simulink model "DecentralizedLFADRC"  (R2018a)
settings: Solver=ode4  StartTime=0.0  StopTime=480  FixedStep=1e-3  MaxStep=1e-4  RelTol=1e-3  EnableMultiTasking=on
values from neighbouring files (symbols this model uses):
  a_1 = 0.5    [DecentralizedADRC.m]
  a_10 = 0.125    [DecentralizedADRC.m]
  a_2 = 0.125    [DecentralizedADRC.m]
  a_3 = 0.125    [DecentralizedADRC.m]
  a_4 = 0.5    [DecentralizedADRC.m]
  a_5 = 0.1    [DecentralizedADRC.m]
  a_6 = 0.1    [DecentralizedADRC.m]
  a_7 = 0.1    [DecentralizedADRC.m]
  a_8 = 0.125    [DecentralizedADRC.m]
  a_9 = 0.5    [DecentralizedADRC.m]
  a_PV1 = 0.125    [DecentralizedADRC.m]
  a_PV2 = 0.2    [DecentralizedADRC.m]
  a_PV3 = 0.125    [DecentralizedADRC.m]
  a_WT1 = 0.125    [DecentralizedADRC.m]
  a_WT3 = 0.125    [DecentralizedADRC.m]
  B1 = (1/Req1)+D    [DecentralizedADRC.m]
  B2 = (1/Req2)+D    [DecentralizedADRC.m]
  B3 = (1/Req3)+D    [DecentralizedADRC.m]
  D = 2    [DecentralizedADRC.m]
  H_A1 = (H1*S1+H2*S2+H3*S3)/(S1+S2+S3)    (= 2.58715528865)    [DecentralizedADRC.m]
  H_A2 = (H4*S4+H5*S5+H6*S6+H7*S7)/(S4+S5+S6+S7)    (= 2.6419)    [DecentralizedADRC.m]
  H_A3 = (H8*S8+H9*S9+H10*S10)/(S8+S9+S10)    (= 2.49952427226)    [DecentralizedADRC.m]
  K1 = -K1    [DecentralizedADRC.m]
  K2 = -K2    [DecentralizedADRC.m]
  K3 = -K3    [DecentralizedADRC.m]
  kpc = 0.8    [DecentralizedADRC.m]
  R1 = 0.0548    [DecentralizedADRC.m]
  R4 = 0.06    [DecentralizedADRC.m]
  R9 = 0.0548    [DecentralizedADRC.m]
  Rp10 = 0.06    [DecentralizedADRC.m]
  Rp2 = 0.06    [DecentralizedADRC.m]
  Rp3 = 0.06    [DecentralizedADRC.m]
  Rp5 = 0.0548    [DecentralizedADRC.m]
  Rp6 = 0.06    [DecentralizedADRC.m]
  Rp7 = 0.06    [DecentralizedADRC.m]
  Rp8 = 0.06    [DecentralizedADRC.m]
  RPV1 = 0.05    [DecentralizedADRC.m]
  RPV2 = 0.05    [DecentralizedADRC.m]
  RPV3 = 0.05    [DecentralizedADRC.m]
  RWT1 = 0.024    [DecentralizedADRC.m]
  RWT3 = 0.024    [DecentralizedADRC.m]
  T12 = 2.5    [DecentralizedADRC.m]
  T13 = 5.0    (= 5)    [DecentralizedADRC.m]
  T23 = 3.8    [DecentralizedADRC.m]
undefined symbols (not defined in the file or in its folder): A_obs_1, A_obs_2, A_obs_3, B_obs_1, B_obs_2, B_obs_3, C_obs_1, C_obs_2, C_obs_3, D_obs_1, D_obs_2, D_obs_3, X_hat_1, X_hat_2, X_hat_3, Xi_hat_1, Xi_hat_2, Xi_hat_3
libraries: cstblocks x94, simulink x40
(part 2 of 2)

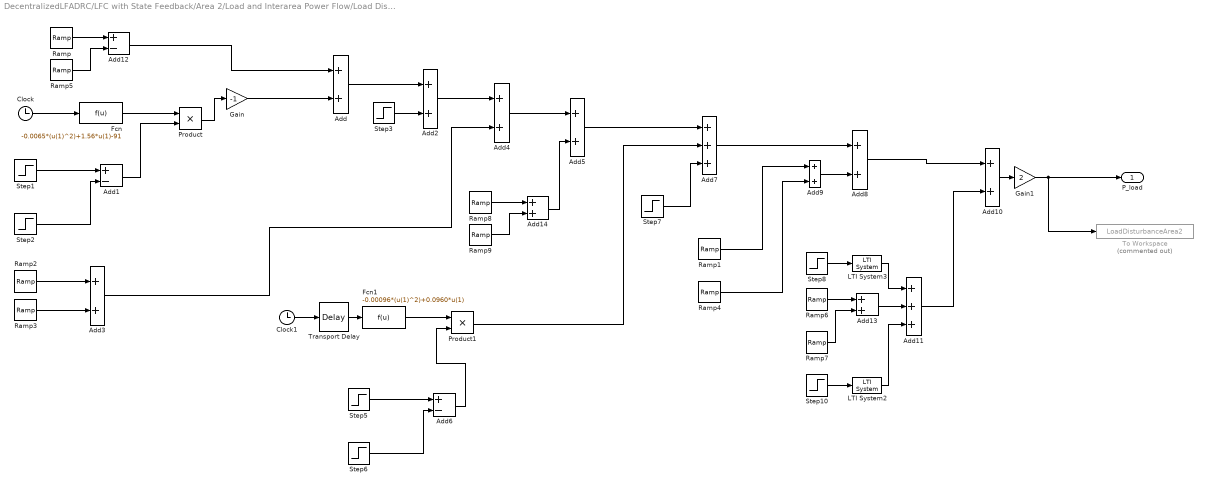
== system DecentralizedLFADRC/LFC with State Feedback/Area 2/Load and Interarea Power Flow/Load Disturbance Area 2  ==
  Add{,2..5,8..10,13..14} (10 alike) : Sum
  Add1 : Sum  Inputs=+-
  Add11 : Sum  Inputs=+++
  Add12 : Sum  Inputs=+-
  Add6 : Sum  Inputs=+-
  Add7 : Sum  Inputs=+++
  Clock : Clock
  Clock1 : Clock
  Fcn : Fcn  Expr=-0.0065*(u(1)^2)+1.56*u(1)-91
  Fcn1 : Fcn  Expr=-0.00096*(u(1)^2)+0.0960*u(1)
  Gain : Gain  Gain=-1
  Gain1 : Gain  Gain=2
  LTI System2 : cstblocks/LTI System  sys=tf(100,conv([1 10],[1 10]))  IC=[]
  LTI System3 : cstblocks/LTI System  sys=tf(100,conv([1 10],[1 10]))  IC=[]
  Product : Product
  Product1 : Product
  Ramp : simulink/Sources/Ramp  slope=1.3  start=10  InitialOutput=0
  Ramp1 : simulink/Sources/Ramp  slope=-0.06  start=340  InitialOutput=0
  Ramp2 : simulink/Sources/Ramp  slope=0.025  start=150  InitialOutput=0
  Ramp3 : simulink/Sources/Ramp  slope=-0.025  start=210  InitialOutput=0
  Ramp4 : simulink/Sources/Ramp  slope=0.06  start=380  InitialOutput=0
  Ramp5 : simulink/Sources/Ramp  slope=1.3  start=12  InitialOutput=0
  Ramp6 : simulink/Sources/Ramp  slope=2.3/10  start=440  InitialOutput=0
  Ramp7 : simulink/Sources/Ramp  slope=-2.3/10  start=450  InitialOutput=0
  Ramp8 : simulink/Sources/Ramp  slope=-1.5/0.5  start=240  InitialOutput=0
  Ramp9 : simulink/Sources/Ramp  slope=1.5/0.5  start=240.5  InitialOutput=0
  Step1 : Step  Time=100  SampleTime=0
  Step10 : Step  Time=450  After=-3.5  SampleTime=0
  Step2 : Step  Time=120  SampleTime=0
  Step3 : Step  Time=120  After=-2.6  SampleTime=0
  Step5 : Step  Time=290  SampleTime=0
  Step6 : Step  Time=340  SampleTime=0
  Step7 : Step  Time=340  After=2.4  SampleTime=0
  Step8 : Step  Time=420  After=1.2  SampleTime=0
  To Workspace : ToWorkspace  Commented=on  VariableName=LoadDisturbanceArea2  SaveFormat=Structure With Time  SampleTime=-1
  Transport Delay : TransportDelay  DelayTime=290
  P_load : Outport
  wires:
  Add10/1 -> Gain1/1
  Clock1/1 -> Transport Delay/1
  Fcn1/1 -> Product1/1
  Add/1 -> Add2/1
  Step3/1 -> Add2/2
  Add5/1 -> Add7/1
  Add2/1 -> Add4/1
  LTI System2/1 -> Add11/3
  Add8/1 -> Add10/1
  Product/1 -> Gain/1
  Add1/1 -> Product/2
  Fcn/1 -> Product/1
  Transport Delay/1 -> Fcn1/1
  Step6/1 -> Add6/2
  Ramp3/1 -> Add3/2
  Clock/1 -> Fcn/1
  Ramp4/1 -> Add9/2
  Step5/1 -> Add6/1
  Step8/1 -> LTI System3/1
  Step1/1 -> Add1/1
  Product1/1 -> Add7/2
  Add6/1 -> Product1/2
  Step10/1 -> LTI System2/1
  LTI System3/1 -> Add11/1
  Step2/1 -> Add1/2
  Step7/1 -> Add7/3
  Ramp2/1 -> Add3/1
  Add9/1 -> Add8/2
  Gain/1 -> Add/2
  Add11/1 -> Add10/2
  Ramp1/1 -> Add9/1
  Add3/1 -> Add4/2
  Add7/1 -> Add8/1
  Add4/1 -> Add5/1
  Gain1/1 -> P_load/1, To Workspace/1
  Ramp/1 -> Add12/1
  Ramp5/1 -> Add12/2
  Add12/1 -> Add/1
  Ramp6/1 -> Add13/1
  Ramp7/1 -> Add13/2
  Add13/1 -> Add11/2
  Ramp9/1 -> Add14/2
  Ramp8/1 -> Add14/1
  Add14/1 -> Add5/2

== system DecentralizedLFADRC/LFC with State Feedback/Area 2/Load and Interarea Power Flow/PV Negative Load Area 2 ==
  Irradiance : Inport
  PV Generator as Negative Load : cstblocks/LTI System  sys=Gpv_load_1  IC=[]
  P_pv : Outport
  wires:
  Irradiance/1 -> PV Generator as Negative Load/1
  PV Generator as Negative Load/1 -> P_pv/1

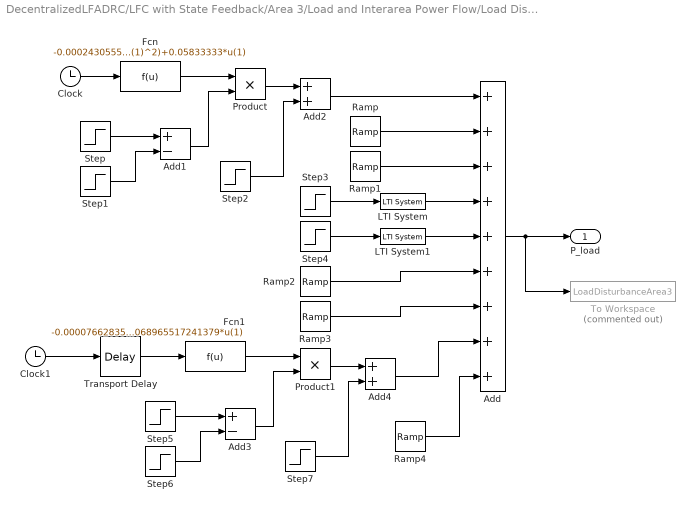
== system DecentralizedLFADRC/LFC with State Feedback/Area 3/Load and Interarea Power Flow/Load Disturbance Area 3  ==
  Add : Sum  Inputs=+++++++++
  Add1 : Sum  Inputs=+-
  Add2 : Sum
  Add3 : Sum  Inputs=+-
  Add4 : Sum
  Clock : Clock
  Clock1 : Clock
  Fcn : Fcn  Expr=-0.000243055555556*(u(1)^2)+0.05833333*u(1)
  Fcn1 : Fcn  Expr=-0.000076628352490*(u(1)^2)+0.068965517241379*u(1)
  LTI System : cstblocks/LTI System  sys=tf(100,conv([1 10],[1 10]))  IC=[]
  LTI System1 : cstblocks/LTI System  sys=tf(100,conv([1 10],[1 10]))  IC=[]
  Product : Product
  Product1 : Product
  Ramp : simulink/Sources/Ramp  slope=-0.1  start=180  InitialOutput=0
  Ramp1 : simulink/Sources/Ramp  slope=0.1  start=215  InitialOutput=0
  Ramp2 : simulink/Sources/Ramp  slope=-0.045  start=330  InitialOutput=0
  Ramp3 : simulink/Sources/Ramp  slope=0.045  start=380  InitialOutput=0
  Ramp4 : simulink/Sources/Ramp  slope=-2/30  start=450  InitialOutput=0
  Step : Step  Time=0  SampleTime=0
  Step1 : Step  Time=120  SampleTime=0
  Step2 : Step  Time=120  After=3.5  SampleTime=0
  Step3 : Step  Time=260  SampleTime=0
  Step4 : Step  Time=300  After=1.25  SampleTime=0
  Step5 : Step  Time=420  SampleTime=0
  Step6 : Step  Time=450  SampleTime=0
  Step7 : Step  Time=450  After=2  SampleTime=0
  To Workspace : ToWorkspace  Commented=on  VariableName=LoadDisturbanceArea3  SaveFormat=Structure With Time  SampleTime=-1
  Transport Delay : TransportDelay  DelayTime=420
  P_load : Outport
  wires:
  Ramp/1 -> Add/2
  Clock/1 -> Fcn/1
  Ramp3/1 -> Add/7
  Step4/1 -> LTI System1/1
  Transport Delay/1 -> Fcn1/1
  Ramp2/1 -> Add/6
  Product/1 -> Add2/1
  Step/1 -> Add1/1
  Add2/1 -> Add/1
  LTI System1/1 -> Add/5
  Step3/1 -> LTI System/1
  Add/1 -> To Workspace/1, P_load/1
  Step2/1 -> Add2/2
  Add1/1 -> Product/2
  Fcn/1 -> Product/1
  Clock1/1 -> Transport Delay/1
  Ramp1/1 -> Add/3
  Step1/1 -> Add1/2
  Step6/1 -> Add3/2
  Step5/1 -> Add3/1
  LTI System/1 -> Add/4
  Ramp4/1 -> Add/9
  Product1/1 -> Add4/1
  Add3/1 -> Product1/2
  Fcn1/1 -> Product1/1
  Step7/1 -> Add4/2
  Add4/1 -> Add/8

== system DecentralizedLFADRC/LFC with State Feedback/Area 3/Load and Interarea Power Flow/PV Negative Load Area 3 ==
  Irradiance : Inport
  PV Generator as Negative Load : cstblocks/LTI System  sys=Gpv_load_1  IC=[]
  P_pv : Outport
  wires:
  Irradiance/1 -> PV Generator as Negative Load/1
  PV Generator as Negative Load/1 -> P_pv/1

== system DecentralizedLFADRC/LFC with ADRC/Area 1/Load and Interarea Power Flow/Load Disturbance Area 1  ==
  Add : Sum  Inputs=+++-+++
  Add1 : Sum  Inputs=+-
  Add2 : Sum
  Add3 : Sum  Inputs=+++
  Clock : Clock
  Fcn : Fcn  Expr=-0.0025*(u(1)^2)+0.2*u(1)
  LTI System : cstblocks/LTI System  sys=tf(100,conv([1 10],[1 10]))  IC=[]
  LTI System1 : cstblocks/LTI System  sys=tf(100,conv([1 10],[1 10]))  IC=[]
  LTI System2 : cstblocks/LTI System  sys=tf(100,conv([1 10],[1 10]))  IC=[]
  Product : Product
  Ramp : simulink/Sources/Ramp  slope=0.05  start=30  InitialOutput=0
  Ramp1 : simulink/Sources/Ramp  slope=-0.05  start=90  InitialOutput=0
  Ramp2 : simulink/Sources/Ramp  slope=0.1  start=300  InitialOutput=0
  Ramp3 : simulink/Sources/Ramp  slope=-0.2  start=330  InitialOutput=0
  Ramp4 : simulink/Sources/Ramp  slope=0.1  start=360  InitialOutput=0
  Step : Step  Time=120  SampleTime=0
  Step1 : Step  Time=180  SampleTime=0
  Step2 : Step  Time=220  SampleTime=0
  Step3 : Step  Time=220  After=4  SampleTime=0
  Step4 : Step  Time=410  After=4  SampleTime=0
  Step5 : Step  Time=450  After=-4  SampleTime=0
  To Workspace : ToWorkspace  VariableName=LoadDisturbanceArea1  SaveFormat=Structure With Time  SampleTime=-1
  Transport Delay : TransportDelay  DelayTime=180
  P_load : Outport
  wires:
  Fcn/1 -> Product/1
  Clock/1 -> Transport Delay/1
  Add/1 -> P_load/1, To Workspace/1
  Transport Delay/1 -> Fcn/1
  Step4/1 -> LTI System1/1
  Ramp/1 -> Add/1
  Ramp4/1 -> Add3/3
  Step5/1 -> LTI System2/1
  Ramp3/1 -> Add3/2
  Step/1 -> LTI System/1
  Product/1 -> Add2/1
  Ramp1/1 -> Add/2
  LTI System/1 -> Add/3
  Step3/1 -> Add2/2
  LTI System2/1 -> Add/7
  Step2/1 -> Add1/2
  LTI System1/1 -> Add/6
  Add1/1 -> Product/2
  Step1/1 -> Add1/1
  Ramp2/1 -> Add3/1
  Add2/1 -> Add/4
  Add3/1 -> Add/5

== system DecentralizedLFADRC/LFC with ADRC/Area 1/Load and Interarea Power Flow/PV Negative Load Area 1 ==
  Irradiance : Inport
  PV Generator as Negative Load : cstblocks/LTI System  sys=Gpv_load_1  IC=[]
  P_pv : Outport
  wires:
  PV Generator as Negative Load/1 -> P_pv/1
  Irradiance/1 -> PV Generator as Negative Load/1

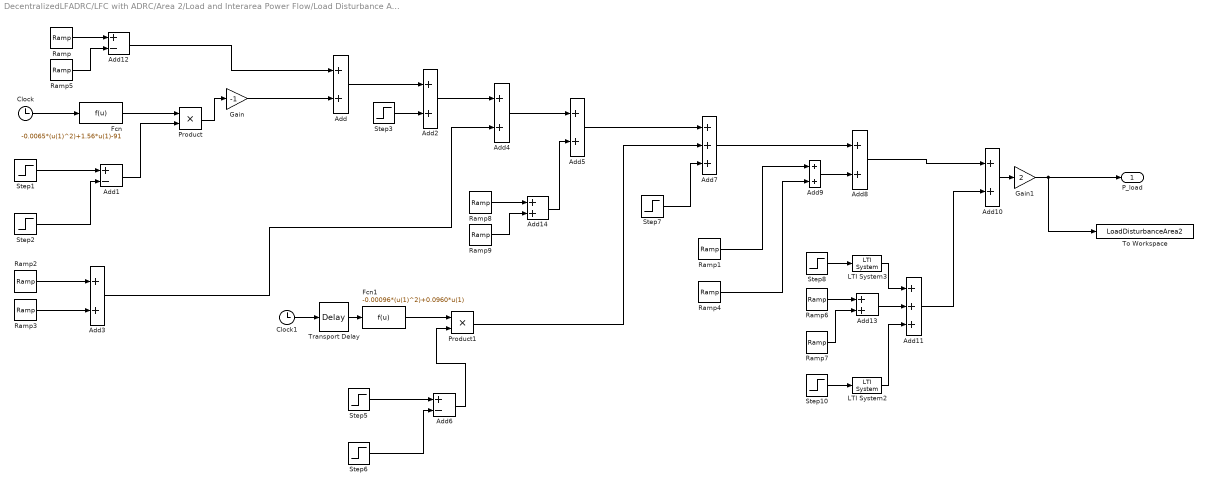
== system DecentralizedLFADRC/LFC with ADRC/Area 2/Load and Interarea Power Flow/Load Disturbance Area 2  ==
  Add{,2..5,8..10,13..14} (10 alike) : Sum
  Add1 : Sum  Inputs=+-
  Add11 : Sum  Inputs=+++
  Add12 : Sum  Inputs=+-
  Add6 : Sum  Inputs=+-
  Add7 : Sum  Inputs=+++
  Clock : Clock
  Clock1 : Clock
  Fcn : Fcn  Expr=-0.0065*(u(1)^2)+1.56*u(1)-91
  Fcn1 : Fcn  Expr=-0.00096*(u(1)^2)+0.0960*u(1)
  Gain : Gain  Gain=-1
  Gain1 : Gain  Gain=2
  LTI System2 : cstblocks/LTI System  sys=tf(100,conv([1 10],[1 10]))  IC=[]
  LTI System3 : cstblocks/LTI System  sys=tf(100,conv([1 10],[1 10]))  IC=[]
  Product : Product
  Product1 : Product
  Ramp : simulink/Sources/Ramp  slope=1.3  start=10  InitialOutput=0
  Ramp1 : simulink/Sources/Ramp  slope=-0.06  start=340  InitialOutput=0
  Ramp2 : simulink/Sources/Ramp  slope=0.025  start=150  InitialOutput=0
  Ramp3 : simulink/Sources/Ramp  slope=-0.025  start=210  InitialOutput=0
  Ramp4 : simulink/Sources/Ramp  slope=0.06  start=380  InitialOutput=0
  Ramp5 : simulink/Sources/Ramp  slope=1.3  start=12  InitialOutput=0
  Ramp6 : simulink/Sources/Ramp  slope=2.3/10  start=440  InitialOutput=0
  Ramp7 : simulink/Sources/Ramp  slope=-2.3/10  start=450  InitialOutput=0
  Ramp8 : simulink/Sources/Ramp  slope=-1.5/0.5  start=240  InitialOutput=0
  Ramp9 : simulink/Sources/Ramp  slope=1.5/0.5  start=240.5  InitialOutput=0
  Step1 : Step  Time=100  SampleTime=0
  Step10 : Step  Time=450  After=-3.5  SampleTime=0
  Step2 : Step  Time=120  SampleTime=0
  Step3 : Step  Time=120  After=-2.6  SampleTime=0
  Step5 : Step  Time=290  SampleTime=0
  Step6 : Step  Time=340  SampleTime=0
  Step7 : Step  Time=340  After=2.4  SampleTime=0
  Step8 : Step  Time=420  After=1.2  SampleTime=0
  To Workspace : ToWorkspace  VariableName=LoadDisturbanceArea2  SaveFormat=Structure With Time  SampleTime=-1
  Transport Delay : TransportDelay  DelayTime=290
  P_load : Outport
  wires:
  Add14/1 -> Add5/2
  Ramp8/1 -> Add14/1
  Ramp9/1 -> Add14/2
  Add13/1 -> Add11/2
  Ramp7/1 -> Add13/2
  Ramp6/1 -> Add13/1
  Add12/1 -> Add/1
  Ramp5/1 -> Add12/2
  Ramp/1 -> Add12/1
  Gain1/1 -> To Workspace/1, P_load/1
  Add4/1 -> Add5/1
  Add7/1 -> Add8/1
  Add3/1 -> Add4/2
  Ramp1/1 -> Add9/1
  Add11/1 -> Add10/2
  Gain/1 -> Add/2
  Add9/1 -> Add8/2
  Ramp2/1 -> Add3/1
  Step7/1 -> Add7/3
  Step2/1 -> Add1/2
  LTI System3/1 -> Add11/1
  Step10/1 -> LTI System2/1
  Add6/1 -> Product1/2
  Product1/1 -> Add7/2
  Step1/1 -> Add1/1
  Step8/1 -> LTI System3/1
  Step5/1 -> Add6/1
  Ramp4/1 -> Add9/2
  Clock/1 -> Fcn/1
  Ramp3/1 -> Add3/2
  Step6/1 -> Add6/2
  Transport Delay/1 -> Fcn1/1
  Fcn/1 -> Product/1
  Add1/1 -> Product/2
  Product/1 -> Gain/1
  Add8/1 -> Add10/1
  LTI System2/1 -> Add11/3
  Add2/1 -> Add4/1
  Add5/1 -> Add7/1
  Step3/1 -> Add2/2
  Add/1 -> Add2/1
  Fcn1/1 -> Product1/1
  Clock1/1 -> Transport Delay/1
  Add10/1 -> Gain1/1

== system DecentralizedLFADRC/LFC with ADRC/Area 2/Load and Interarea Power Flow/PV Negative Load Area 2 ==
  Irradiance : Inport
  PV Generator as Negative Load : cstblocks/LTI System  sys=Gpv_load_1  IC=[]
  P_pv : Outport
  wires:
  PV Generator as Negative Load/1 -> P_pv/1
  Irradiance/1 -> PV Generator as Negative Load/1

== system DecentralizedLFADRC/LFC with ADRC/Area 3/Load and Interarea Power Flow/Load Disturbance Area 3  ==
  Add : Sum  Inputs=+++++++++
  Add1 : Sum  Inputs=+-
  Add2 : Sum
  Add3 : Sum  Inputs=+-
  Add4 : Sum
  Clock : Clock
  Clock1 : Clock
  Fcn : Fcn  Expr=-0.000243055555556*(u(1)^2)+0.05833333*u(1)
  Fcn1 : Fcn  Expr=-0.000076628352490*(u(1)^2)+0.068965517241379*u(1)
  LTI System : cstblocks/LTI System  sys=tf(100,conv([1 10],[1 10]))  IC=[]
  LTI System1 : cstblocks/LTI System  sys=tf(100,conv([1 10],[1 10]))  IC=[]
  Product : Product
  Product1 : Product
  Ramp : simulink/Sources/Ramp  slope=-0.1  start=180  InitialOutput=0
  Ramp1 : simulink/Sources/Ramp  slope=0.1  start=215  InitialOutput=0
  Ramp2 : simulink/Sources/Ramp  slope=-0.045  start=330  InitialOutput=0
  Ramp3 : simulink/Sources/Ramp  slope=0.045  start=380  InitialOutput=0
  Ramp4 : simulink/Sources/Ramp  slope=-2/30  start=450  InitialOutput=0
  Step : Step  Time=0  SampleTime=0
  Step1 : Step  Time=120  SampleTime=0
  Step2 : Step  Time=120  After=3.5  SampleTime=0
  Step3 : Step  Time=260  SampleTime=0
  Step4 : Step  Time=300  After=1.25  SampleTime=0
  Step5 : Step  Time=420  SampleTime=0
  Step6 : Step  Time=450  SampleTime=0
  Step7 : Step  Time=450  After=2  SampleTime=0
  To Workspace : ToWorkspace  VariableName=LoadDisturbanceArea3  SaveFormat=Structure With Time  SampleTime=-1
  Transport Delay : TransportDelay  DelayTime=420
  P_load : Outport
  wires:
  Add4/1 -> Add/8
  Step7/1 -> Add4/2
  Fcn1/1 -> Product1/1
  Add3/1 -> Product1/2
  Product1/1 -> Add4/1
  Ramp4/1 -> Add/9
  LTI System/1 -> Add/4
  Step5/1 -> Add3/1
  Step6/1 -> Add3/2
  Step1/1 -> Add1/2
  Ramp1/1 -> Add/3
  Clock1/1 -> Transport Delay/1
  Fcn/1 -> Product/1
  Add1/1 -> Product/2
  Step2/1 -> Add2/2
  Add/1 -> P_load/1, To Workspace/1
  Step3/1 -> LTI System/1
  LTI System1/1 -> Add/5
  Add2/1 -> Add/1
  Step/1 -> Add1/1
  Product/1 -> Add2/1
  Ramp2/1 -> Add/6
  Transport Delay/1 -> Fcn1/1
  Step4/1 -> LTI System1/1
  Ramp3/1 -> Add/7
  Clock/1 -> Fcn/1
  Ramp/1 -> Add/2

== system DecentralizedLFADRC/LFC with ADRC/Area 3/Load and Interarea Power Flow/PV Negative Load Area 3 ==
  Irradiance : Inport
  PV Generator as Negative Load : cstblocks/LTI System  sys=Gpv_load_1  IC=[]
  P_pv : Outport
  wires:
  PV Generator as Negative Load/1 -> P_pv/1
  Irradiance/1 -> PV Generator as Negative Load/1
